simulink model "smdik"  (R2016a)
settings: Solver=FixedStepDiscrete  StartTime=0.0  StopTime=10.0  FixedStep=0.1  RelTol=1e-3
settings Model: Creator=Samvrit  LastModifiedBy=Samvrit
settings SolverCC: AutoInsertRateTranBlk=on
settings DataIOCC: LimitDataPoints=on
settings DebuggingCC: AllowSymbolicDim=off
settings ConfigComp: CovModelRefEnable=Off  CovSFcnEnable=off

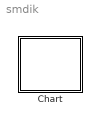
== system smdik ==
  Chart : Stateflow chart  TreatAsAtomicUnit=on

== stateflow chart smdik/Chart ==
  state IDLE
  state CALCULATE_ROTATION_MATRIX
    entry: using x,y,z,order
  state CALCULATE_JOINT_ANGLES
    entry: using rotmatrix
  state SIMULATE_ROBOT
    entry: using jointangles
  (default) -> IDLE
  IDLE -> CALCULATE_ROTATION_MATRIX [order 1] : compute_button_press
  CALCULATE_ROTATION_MATRIX -> IDLE : rotation_matrix_creation
  IDLE -> CALCULATE_JOINT_ANGLES [order 2] : jointangles_button_press
  CALCULATE_JOINT_ANGLES -> IDLE : joint_angle_calculation
  IDLE -> SIMULATE_ROBOT [order 3] : simulate_button_press
  SIMULATE_ROBOT -> IDLE : simulation_completion
